simulink library "DelayLibraryBtc"  (R2022b)
settings: Solver=VariableStepAuto  StartTime=0.0  StopTime=10.0  RelTol=1e-3
undefined symbols (not defined in the file or in its folder): Row
libraries: HandyTextFile x6, AudioStats x4, FeaturePath x3, ITC x2, TuneVar x2, CapturedConstLib x1, TOP x1, RTC x1, $bdroot x1
settings Model: Creator=sd49596  LastModifiedBy=jz1055514
settings SolverCC: AlgebraicLoopSolver=TrustRegion
settings DebuggingCC: UnconnectedInputMsg=warning  UnconnectedOutputMsg=warning  UnconnectedLineMsg=warning  SFMachineParentedDataDiag=warning
settings ModelReferenceCC: EnableRefExpFcnMdlSchedulingChecks=on

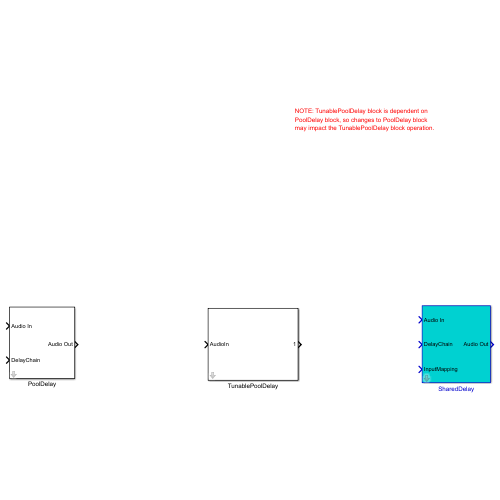
[thumbnail: Simulink's stored preview of the top-level diagram]
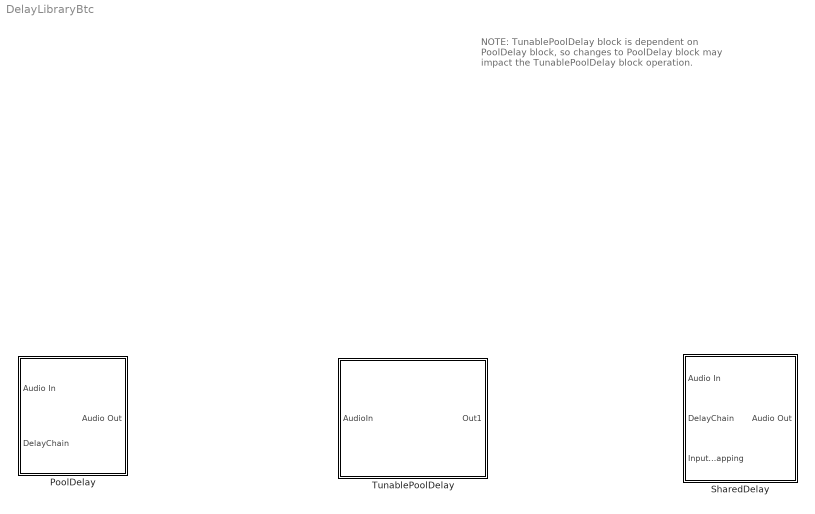
== system DelayLibraryBtc ==
  note: NOTE: TunablePoolDelay block is dependent on
      | PoolDelay block, so changes to PoolDelay block
      | may impact the TunablePoolDelay block operation.
  PoolDelay : Subsystem  mask(Bose Pool Delay){Config=[]}
      mask prompts: Config "PoolDelayConfig"
      mask help:
      | Pool Delay is a multi-channel delay module with one single delay pool and adjustable delays per channel.  It provides support for delays greater than or equal to zero for one or more channels.  Total delay buffer size is the sum of all channel delays.  The Pool Delay model supports three different implementations, selectable from the model mask:
      |
      | - L1 Memory:  Optimized CRL (Code Replacement Library) code running on core with delay buffer in L1 Memory
      | - L2 Memory:  Optimized CRL code running on core and using DMA for memory copies with primary delay buffer in L2 or L3 Memory
      | - Generic:  Generic Matlab implementation running on core for targets without CRL support
      |
      | This model has two inputs and one output:
      |
      | - AudioIn [in]:  Audio input stream containing audio frame samples for one or more channels  [frameSize x numChannels]
      | - Delay [in]:  Delay in samples for each channel  [1 x numChannels]
      | - AudioOut [out]:  Audio output stream containing delayed audio frame samples for one or more channels  [frameSize x numChannels]
      |
      | NOTE: The Pool Delay codeWorkMemory buffer should always be mapped to L1 memory or core MIPS usage will increase.
      |
      | For more information, please see 'Help'.
      mask init:
      | blkh=gcbh;
      | Config=BTConfig.Assert(blkh,Config);
      | 
      | Config.Validate();
      | Config.DoMaskInit(blkh);
      mask Help:
      | Help on Mask Parameters:
      | 
      | All variants of the model contain the following mask parameters:
      | - Implementation:  Selects the desired model implementation to use (L1 Memory, L2 Memory, or Generic)
      | - Total Allotted Delay:  The provides delay buffer sizing for the maximum Room Model Down Load (RMDL) or non-RMDL delay configuration required.  It is the sum of all channels delays in samples for the largest RMDL delay case.  (scalar)
      | - Frame Size:  Specifies the audio frame size in samples (scalar)
      | - Number Channels:  Specifies the number of channel and applies to the audio input, output, and delay channels (scalar)
      | 
      | The 'L2 Memory' implementation contains the following additional mask parameter:
      | 
      | - Delay Sizes Required: The appropriate check boxes must be checked to specify delay categories required.  Delay categories include the following: (delays <= frameSize), (frameSize < delays < (2 * frameSize)), and (delays >= (2 * frameSize).  The correct selection of these delay categories is required to ensure the delay buffers and other model data is sized correctly.
      | 
      | Note that since the 'L2 Memory' implementations takes advantage of DMA memory copies performed by the hardware DMA engine, the implementation differs from the other model implementations and in order to minimize the memory usage required to support all channel delay configurations, the channel delay categories required must be known.  The specific delay cases required for RMDL and non-RMDL model instances determine overall memory required for delay buffers and DMA descriptor memory.
      | 
      | Mask Usage Example:
      | 
      | 3 input and output channels, with channel delays of 16, 48, 80 samples for a case that does not require RMDL, and a frame size of 32 samples.
      | 
      | For example, to use the  L1 Memory implementation, set the mask parameters as follows:
      | 
      | Implementation = 'L1 Memory'
      | Total RMDL Allotted Delay = 144        (16 + 48 + 80)
      | Frame Size = 32
      | Number Channels = 3
      | 
      | For the same example with the L2 Memory implementation, set all the above parameters as stated, except with:
      | 
      | Implementation = 'L2 Memory'
      | Delay Sizes Required should have all delay categories checked, as the delays of 16, 48, 80 include all categories.  These parameters and the Total Allotted Delay are used to size memory to support the delay configuration.  If for example, all delays required were less than equal to a frame only that delay category should be checked.
      | 
      | Note that 'Delay Sizes Required' is specific to the L2 Memory implementation and does not apply to the other implementations.
      | 
      | The 'Generic' implementation would require the identical mask parameter initialization as the L1 memory implementation, except with:
      | 
      | Implementation = 'Generic'
  SharedDelay : Subsystem  mask(Bose Shared Delay){Config=[]}
      mask prompts: Config "SharedDelayConfig"
      mask help:
      | Shared Delay is a multi-input channel delay module with one or more adjustable output delay taps per input channel, based on how input channels are mapped to outputs.  It provides support for delays greater than or equal to zero.  The Shared Delay model supports only one implementation.  It is a DMA based write before delay buffer read implementation, with total delay buffer size of the sum of the maximum output channel tap delay for each input channel, plus one frame size per input channel.
      |
      | This model has two inputs and one output:
      |
      | - AudioIn [in]:  Audio input stream containing audio frame samples for one or more input channels  [frameSize x numInputs]
      | - DelayChain [in]:  Delay in samples for all input channel's output tap channels  [1 x numOutputs]
      | - InputMapping [in]:  Zero based mapping of input channels to output tap channels  [1 x numOutputs]
      | - AudioOut [out]:  Audio output stream containing delayed audio frame samples for one or more output channels  [frameSize x numOutputs]
      |
      | The delay buffer can be mapped to L2 or L3 memory with proper definition of the code generated pragma section memory mappings.
      |
      | NOTE: The Shared Delay codeWorkMemory buffer should always be mapped to L1 memory or core MIPS usage will increase.
      |
      | For more information, please see 'Help'.
      mask init:
      | blkh=gcbh;
      | Config=BTConfig.Assert(blkh,Config);
      | % Validate mask settings
      | Config.Validate();
      | Config.DoMaskInit(blkh);
      mask Help:
      | Help on Mask Parameters:
      | 
      | The Shared Delay model contains the following mask parameters:
      | 
      | - Total Allotted Delay:  Specifies delay buffer sizing for the maximum Room Model Down Load (RMDL) or non-RMDL delay configuration required.  It is the sum of the maximum output channel tap delay for each input channel in samples that supports the largest RMDL delay case.  (scalar)
      | - Frame Size:  Specifies the audio frame size in samples (scalar)
      | - Number Input Channels:  Specifies the number of input channels and applies to the audio inputs (scalar)
      | - Number Output Channels:  Specifies the number of output channels and applies to the audio outputs, delays and input mapping (scalar)
      | 
      | Mask Usage Example:
      | 
      | 2 input channels, with output channel tap delays of 16, 48, 80 samples for input 1 and output channel tap delays of 37, 62 samples for input channel 2.    Assumption is this case does not require RMDL and the frame size is 32 samples.
      | 
      | For this example, set the mask parameters and inputs as follows:
      | 
      | Total Allotted Delay = 142        max( [16 48 80] ) + max( [37  62] ) = 80 + 62
      | Frame Size = 32
      | Number Inputs = 2
      | Number Outputs = 5                (3 + 2)
      | 
      | DelayChain = [16 48 80 37 62]
      | InputMapping = [0 0 0 1 1]
  TunablePoolDelay : Subsystem  mask{Config=[]}
      mask prompts: Config "TunablePoolDelayConfig"
      mask init:
      | blkh=gcbh;
      | Config=BTConfig.Assert(blkh,Config);
      | 
      | Config.Validate();
      | Config.DoMaskInit(blkh);

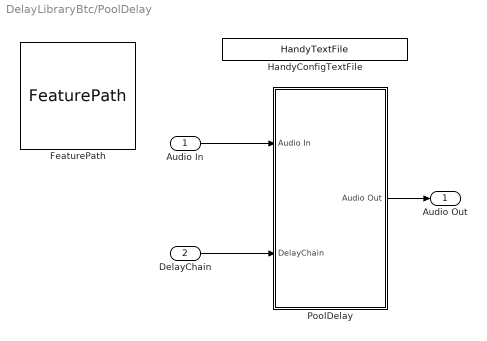
== system DelayLibraryBtc/PoolDelay ==
  Audio In : Inport
  DelayChain : Inport  Port=2  OutDataTypeStr=uint32  PortDimensions=[1, Config.NumChannels]
  FeaturePath : FeaturePath/FeaturePath  FeatureName=PoolDelay  IsGroup=off  GroupNumber=-1  IsModule=off  TriggerInit=[-40 9 75 116]
      settings: SourceProductName=Bose Talaria
  HandyConfigTextFile : HandyTextFile/HandyTextFile  TemplateSource=Config  FileSuffix=File  OpenDialogOnLoad=off  UseThisBlockName=off  AddGrandParentNamePrefix=off  TheDefaultText=% $(FILENAME) $(PREFIX) $(SUFFIX)  ShowInLibBrowser=on
      settings: SourceProductName=Bose Talaria
  PoolDelay : Subsystem  Variant=on
  Audio Out : Outport
  wires:
  Audio In/1 -> PoolDelay/1(Audio In)
  DelayChain/1 -> PoolDelay/2(DelayChain)
  PoolDelay/1(Audio Out) -> Audio Out/1

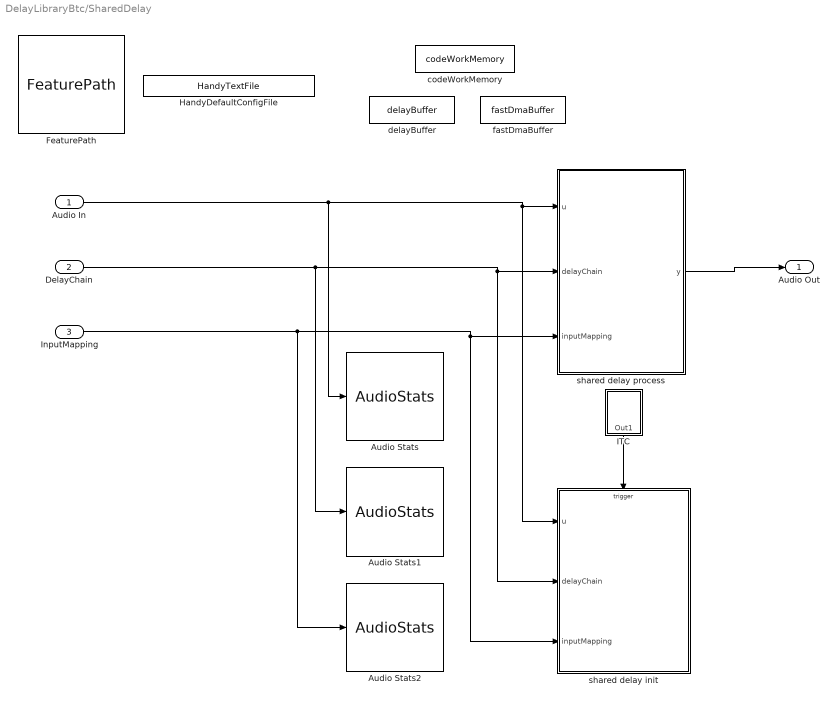
== system DelayLibraryBtc/SharedDelay ==
  Audio In : Inport
  DelayChain : Inport  Port=2  OutDataTypeStr=int32  PortDimensions=[1, Config.NumOutputs]
  InputMapping : Inport  Port=3  OutDataTypeStr=int32  PortDimensions=[1 Config.NumOutputs]
  Audio Stats : AudioStats/AudioStats  DoSampleRate=off  TypeSampleRate=Inherit: auto  DoCallRate=off  TypeCallRate=Inherit: auto  DoFrameSize=off  TypeFrameSize=Inherit: auto  DoChannelCount=off  TypeChannelCount=Inherit: auto  DoTaskRateFactor=off  TypeTaskRateFactor=Inherit: auto  MacroNameRoot=AUDIO  MacroNameRootEval='AUDIO'  IsMacroNameEval=off  MacroSampleRate=off  MacroCallRate=off  MacroFrameSize=off  MacroChannelCount=off  MacroTaskRateFactor=off  MacroTaskId=off  ValidateSampleRate=off  ValueSampleRate=[]  ValidateCallRate=off  ValueCallRate=[]  ValidateFrameSize=on  ValueFrameSize=Config.FrameSize  ValidateChannelCount=on  ValueChannelCount=Config.NumInputs  ValidateTaskRateFactor=off  ValueTaskRateFactor=[]
      settings: SourceProductName=Bose Talaria
  Audio Stats1 : AudioStats/AudioStats  DoSampleRate=off  TypeSampleRate=Inherit: auto  DoCallRate=off  TypeCallRate=Inherit: auto  DoFrameSize=off  TypeFrameSize=Inherit: auto  DoChannelCount=off  TypeChannelCount=Inherit: auto  DoTaskRateFactor=off  TypeTaskRateFactor=Inherit: auto  MacroNameRoot=AUDIO  MacroNameRootEval='AUDIO'  IsMacroNameEval=off  MacroSampleRate=off  MacroCallRate=off  MacroFrameSize=off  MacroChannelCount=off  MacroTaskRateFactor=off  MacroTaskId=off  ValidateSampleRate=off  ValueSampleRate=[]  ValidateCallRate=off  ValueCallRate=[]  ValidateFrameSize=off  ValueFrameSize=[]  ValidateChannelCount=on  ValueChannelCount=Config.NumOutputs  ValidateTaskRateFactor=off  ValueTaskRateFactor=[]
      settings: SourceProductName=Bose Talaria
  Audio Stats2 : AudioStats/AudioStats  DoSampleRate=off  TypeSampleRate=Inherit: auto  DoCallRate=off  TypeCallRate=Inherit: auto  DoFrameSize=off  TypeFrameSize=Inherit: auto  DoChannelCount=off  TypeChannelCount=Inherit: auto  DoTaskRateFactor=off  TypeTaskRateFactor=Inherit: auto  MacroNameRoot=AUDIO  MacroNameRootEval='AUDIO'  IsMacroNameEval=off  MacroSampleRate=off  MacroCallRate=off  MacroFrameSize=off  MacroChannelCount=off  MacroTaskRateFactor=off  MacroTaskId=off  ValidateSampleRate=off  ValueSampleRate=[]  ValidateCallRate=off  ValueCallRate=[]  ValidateFrameSize=off  ValueFrameSize=[]  ValidateChannelCount=on  ValueChannelCount=Config.NumOutputs  ValidateTaskRateFactor=off  ValueTaskRateFactor=[]
      settings: SourceProductName=Bose Talaria
  FeaturePath : FeaturePath/FeaturePath  FeatureName=SharedDelay  IsGroup=off  GroupNumber=-1  IsModule=off  TriggerInit=[185 -31 300 76]
      settings: SourceProductName=Bose Talaria
  HandyDefaultConfigFile : HandyTextFile/HandyTextFile  TemplateSource=Config  FileSuffix=Init  OpenDialogOnLoad=off  UseThisBlockName=off  AddGrandParentNamePrefix=off  TheDefaultText=|  ShowInLibBrowser=on
      | % $(FILENAME) Setup model parameters for each "Init" callback (e.g. update diagram)
      | sample_rate_in_hertz = 44100;
      | frame_size = 32;
      | sysin_channel_count = 2;
      settings: SourceProductName=Bose Talaria
  ITC : Subsystem  mask(Bose Initialization Trigger Control){}
      mask help: This block emits a function trigger for logic intended to execute at subsystem initialization time. Make sure not to reference any "live" signals
      mask init:
      | CodeID = InitTriggerControlMask.DoInit(gcbh);
      | ok = true;
      mask Display:
      | % retrieve icon definition
      | [path,w,h] = InitTriggerControlMask.Icon();
      | 
      | % retrieve the block's pixel size
      | pos = get(gcbh,'position');
      | bw = pos(3) - pos(1);
      | bh = pos(4) - pos(2);
      | 
      | % draw  icon to the center left
      | xAdj = bw/2 - w/2;
      | yAdj = bh/2 - h/2 + 4;
      | for i=1:length(path)
      |     patch(path(i).x+xAdj, path(i).y+yAdj, path(i).rgb);
      | end
      | 
      | text(bw*0.5, bh*0.2, 'ITC', 'horizontalAlignment', 'center');
      | 
      | % show X on error
      | if (exist('ok','var') && ok)
      | 	patch(0,0,[1 1 1]);
      | 	patch(bw,bh,[1 1 1]);
      | else
      | 	tx=bw*0.03;
      | 	ty=bh*0.03;
      | 	patch([0 tx bw bw-tx], [ty 0 bh-ty bh], [1 0 0]);
      | 	patch([0 bw-tx bw tx], [bh-ty 0 ty bh], [1 0 0]);
      | end
  codeWorkMemory : DataStoreMemory  DataStoreName=codeWorkMemory  WriteAfterWriteMsg=warning  InitialValue=Config.CodeWorkMemoryInitVal  EmbeddedSignalClassName=Blocklib.Signal  ShowAdditionalParam=off  OutDataTypeStr=uint32
  delayBuffer : DataStoreMemory  DataStoreName=delayBuffer  ReadBeforeWriteMsg=warning  WriteAfterWriteMsg=warning  WriteAfterReadMsg=warning  InitialValue=Config.DelayBufferInitVal  EmbeddedSignalClassName=Blocklib.Signal  ShowAdditionalParam=off  OutDataTypeStr=single
  fastDmaBuffer : DataStoreMemory  DataStoreName=fastDmaBuffer  ReadBeforeWriteMsg=warning  WriteAfterWriteMsg=warning  WriteAfterReadMsg=warning  InitialValue=Config.FastDelayBufferInitVal  EmbeddedSignalClassName=Blocklib.Signal  ShowAdditionalParam=off  OutDataTypeStr=single
  shared delay init : MATLAB Function  TreatAsAtomicUnit=on  RTWFcnName=foo
  shared delay process : MATLAB Function  TreatAsAtomicUnit=on
  Audio Out : Outport  VectorParamsAs1DForOutWhenUnconnected=off
  wires:
  Audio In/1 -> shared delay process/1(u), shared delay init/1(u), Audio Stats/1
  InputMapping/1 -> shared delay process/3(inputMapping), shared delay init/3(inputMapping), Audio Stats2/1
  ITC/1(Out1) -> shared delay init/Trigger
  shared delay process/1(y) -> Audio Out/1
  DelayChain/1 -> shared delay process/2(delayChain), shared delay init/2(delayChain), Audio Stats1/1

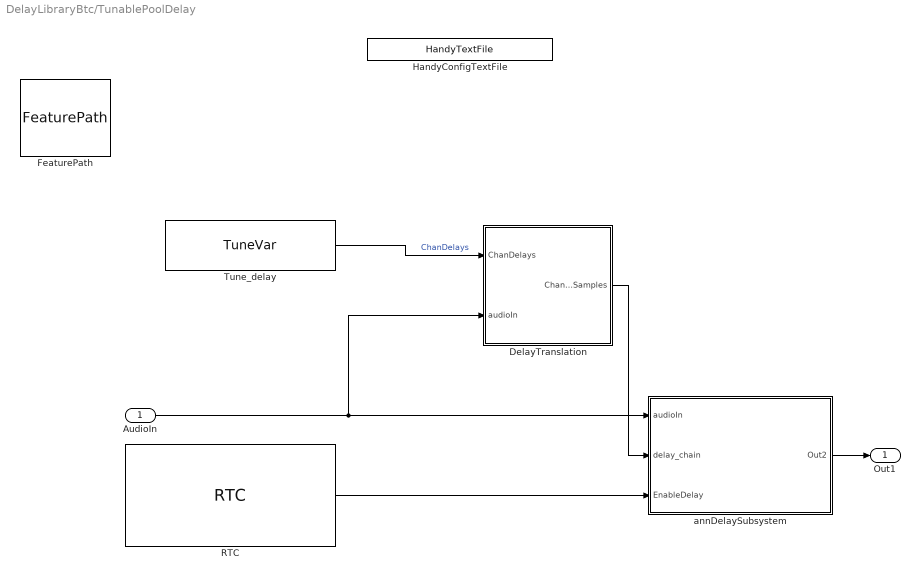
== system DelayLibraryBtc/TunablePoolDelay ==
  AudioIn : Inport
  DelayTranslation : Subsystem  mask{delayType=Config.delayType, maxTotalDelay=Config.MaxTotalDelay}
      mask prompts: delayType "Delay Type"; maxTotalDelay "Max Total Delay"
  FeaturePath : FeaturePath/FeaturePath  FeatureName=TunablePoolDelay  IsGroup=off  GroupNumber=-1  IsModule=off  TriggerInit=[500 209 590 286]
      settings: SourceProductName=Bose Talaria
  HandyConfigTextFile : HandyTextFile/HandyTextFile  TemplateSource=Config  FileSuffix=File  OpenDialogOnLoad=off  UseThisBlockName=off  AddGrandParentNamePrefix=off  TheDefaultText=% $(FILENAME) $(PREFIX) $(SUFFIX)  ShowInLibBrowser=on
      settings: SourceProductName=Bose Talaria
  RTC : RTC/RTC  REQ_Priority=RTC_Mask.NormalPriority  RequestAtInit=off  EnableRequest=off  REQElemName1=Enable_annDelay  REQElemType1=uint32  REQElemWidth1=1  REQElemInitial1=Config.enableDelay  REQElemType2=uint32  REQElemWidth2=1  REQElemInitial2=[]  REQElemType3=uint32  REQElemWidth3=1  REQElemInitial3=[]  REQElemType4=uint32  REQElemWidth4=1  REQElemInitial4=[]  REQElemType5=uint32  REQElemWidth5=1  REQElemInitial5=[]  REQElemType6=uint32  REQElemWidth6=1  REQElemInitial6=[]  REQElemType7=uint32  REQElemWidth7=1  REQElemInitial7=[]  REQElemType8=uint32  REQElemWidth8=1  REQElemInitial8=[]  REQElemType9=uint32  REQElemWidth9=1  REQElemInitial9=[]  REQElemType10=uint32  REQElemWidth10=1  REQElemInitial10=[]  EnableResponse=on  EnableRSP_StatusIn=off  RSPElemType1=uint32  RSPElemWidth1=1  RSPElemType2=uint32  RSPElemWidth2=1  RSPElemType3=uint32  RSPElemWidth3=1  RSPElemType4=uint32  RSPElemWidth4=1  RSPElemType5=uint32  RSPElemWidth5=1  RSPElemType6=uint32  RSPElemWidth6=1  RSPElemType7=uint32  RSPElemWidth7=1  RSPElemType8=uint32  RSPElemWidth8=1  RSPElemType9=uint32  RSPElemWidth9=1  RSPElemType10=uint32  RSPElemWidth10=1  EnableNotification=off  EnableNTF_PrepTrig=off  NTFElemType1=uint32  NTFElemWidth1=1  NTFElemType2=uint32  NTFElemWidth2=1  NTFElemType3=uint32  NTFElemWidth3=1  NTFElemType4=uint32  NTFElemWidth4=1  NTFElemType5=uint32  NTFElemWidth5=1  NTFElemType6=uint32  NTFElemWidth6=1  NTFElemType7=uint32  NTFElemWidth7=1  NTFElemType8=uint32  NTFElemWidth8=1  NTFElemType9=uint32  NTFElemWidth9=1  NTFElemType10=uint32  NTFElemWidth10=1  MaskMessageName=Enable_Delay
      settings: SourceProductName=Bose Talaria
  Tune_delay : TuneVar/TuneVar  TuneName=ChanDelays  SpecifyMaxSize=off  VariableDim=1 (Row)  MaxSize=[1 1]  TunabilityNumber=1  MinValue=[]  MaxValue=[]  TriggerInit=[645 350 815 400]  MaskValue=Config.delayChains
      settings: SourceProductName=Bose Talaria
  annDelaySubsystem : Subsystem
  Out1 : Outport  VectorParamsAs1DForOutWhenUnconnected=off
  wires:
  AudioIn/1 -> DelayTranslation/2(audioIn), annDelaySubsystem/1(audioIn)
  RTC/1 -> annDelaySubsystem/3(EnableDelay)
  Tune_delay/1 -> DelayTranslation/1(ChanDelays)  "ChanDelays"
  annDelaySubsystem/1(Out2) -> Out1/1
  DelayTranslation/1(ChanDelaysSamples) -> annDelaySubsystem/2(delay_chain)

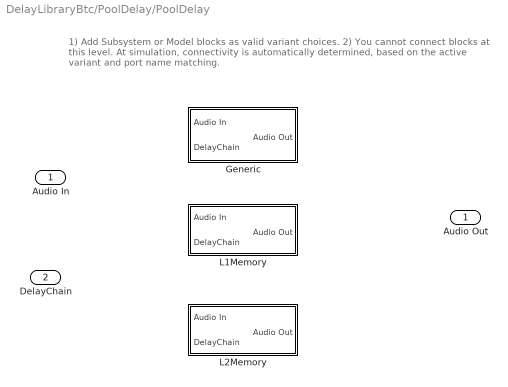
== system DelayLibraryBtc/PoolDelay/PoolDelay ==
  note: 1) Add Subsystem or Model blocks as valid variant choices.
      | 2) You cannot connect blocks at this level. At simulation, connectivity is automatically
      | determined, based on the active variant and port name matching.
  Audio In : Inport
  DelayChain : Inport  Port=2
  Generic : Subsystem  VariantControl=(default)
  L1Memory : Subsystem  VariantControl=Config.Breed == PoolDelayBreedEnum.L1Memory
  L2Memory : Subsystem  VariantControl=Config.Breed == PoolDelayBreedEnum.L2Memory
  Audio Out : Outport

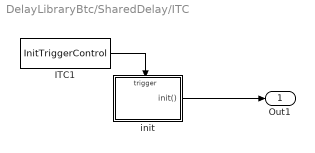
== system DelayLibraryBtc/SharedDelay/ITC ==
  ITC1 : S-Function  FunctionName=InitTriggerControl  Parameters=CodeID, 0  SFunctionDeploymentMode=off  EnableBusSupport=off
  init : MATLAB Function  TreatAsAtomicUnit=on  RTWFcnName=InitTrigger_DelayLibraryBtc_1_62
      settings: RTWSystemCode=Nonreusable function
  Out1 : Outport  VectorParamsAs1DForOutWhenUnconnected=off
  wires:
  init/1(init()) -> Out1/1
  ITC1/1 -> init/Trigger

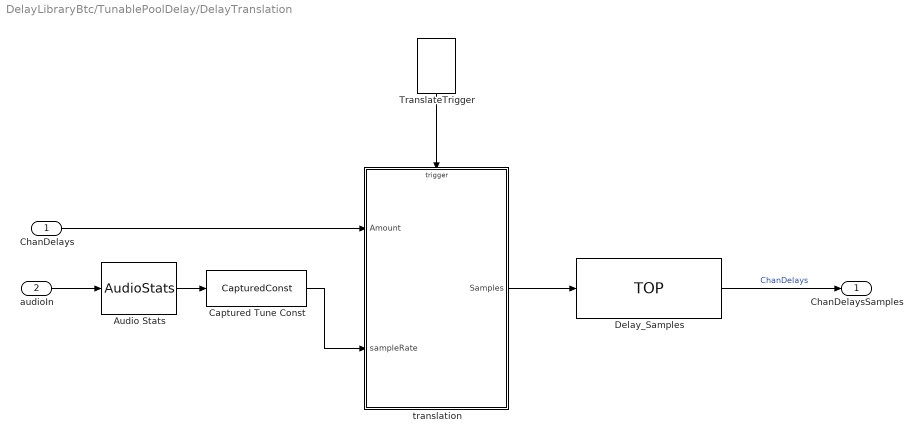
== system DelayLibraryBtc/TunablePoolDelay/DelayTranslation ==
  ChanDelays : Inport
  audioIn : Inport  Port=2
  Audio Stats : AudioStats/AudioStats  DoSampleRate=on  TypeSampleRate=Inherit: auto  DoCallRate=off  TypeCallRate=Inherit: auto  DoFrameSize=off  TypeFrameSize=Inherit: auto  DoChannelCount=off  TypeChannelCount=Inherit: auto  DoTaskRateFactor=off  TypeTaskRateFactor=Inherit: auto  MacroNameRoot=AUDIO  MacroNameRootEval='AUDIO'  IsMacroNameEval=off  MacroSampleRate=off  MacroCallRate=off  MacroFrameSize=off  MacroChannelCount=off  MacroTaskRateFactor=off  MacroTaskId=off  ValidateSampleRate=off  ValueSampleRate=[]  ValidateCallRate=off  ValueCallRate=[]  ValidateFrameSize=off  ValueFrameSize=[]  ValidateChannelCount=off  ValueChannelCount=[]  ValidateTaskRateFactor=off  ValueTaskRateFactor=[]
      settings: SourceProductName=Bose Talaria
  Captured Tune Const : CapturedConstLib/CapturedConst  TriggerInit=[1245 262 1345 298]  Role=Automatic
      settings: SourceProductName=Bose Talaria
  Delay_Samples : TOP/TOP  TriggerInit=[575 240 720 300]  TopName=ChanDelays  DataTypeOut=uint32  BankNumber=0  PreOverlay=false  PostOverlay=Config.PostOverlayRequired  CompatibilityString=[]  Role=Automatic
      settings: SourceProductName=Bose Talaria
  TranslateTrigger : TuneVar/TranslateTrigger  TriggerInit=[1456 30 1494 85]
      settings: SourceProductName=Bose Talaria
  translation : MATLAB Function  TreatAsAtomicUnit=on
  ChanDelaysSamples : Outport  VectorParamsAs1DForOutWhenUnconnected=off
  wires:
  ChanDelays/1 -> translation/1(Amount)
  Audio Stats/1 -> Captured Tune Const/1
  TranslateTrigger/1 -> translation/Trigger
  audioIn/1 -> Audio Stats/1
  Delay_Samples/1 -> ChanDelaysSamples/1  "ChanDelays"
  Captured Tune Const/1 -> translation/2(sampleRate)
  translation/1(Samples) -> Delay_Samples/1

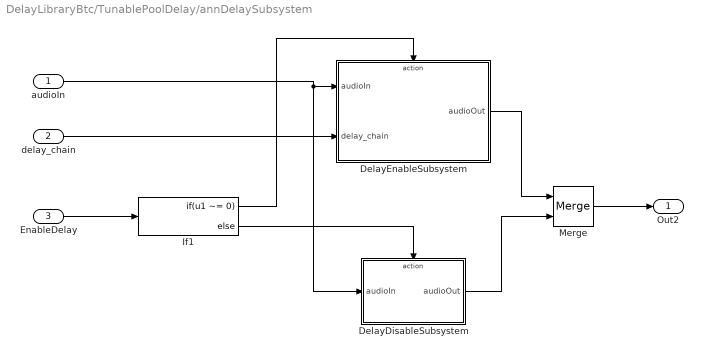
== system DelayLibraryBtc/TunablePoolDelay/annDelaySubsystem ==
  audioIn : Inport
  delay_chain : Inport  Port=2
  EnableDelay : Inport  Port=3
  DelayDisableSubsystem : Subsystem  TreatAsAtomicUnit=on
  DelayEnableSubsystem : Subsystem  TreatAsAtomicUnit=on
  If1 : If  IfExpression=u1 ~= 0
  Merge : Merge
  Out2 : Outport  VectorParamsAs1DForOutWhenUnconnected=off
  wires:
  If1/1 -> DelayEnableSubsystem/Action
  audioIn/1 -> DelayEnableSubsystem/1(audioIn), DelayDisableSubsystem/1(audioIn)
  EnableDelay/1 -> If1/1
  If1/2 -> DelayDisableSubsystem/Action
  DelayEnableSubsystem/1(audioOut) -> Merge/1
  delay_chain/1 -> DelayEnableSubsystem/2(delay_chain)
  DelayDisableSubsystem/1(audioOut) -> Merge/2
  Merge/1 -> Out2/1

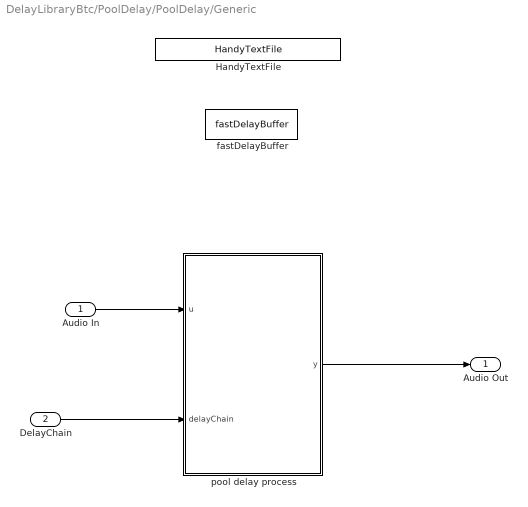
== system DelayLibraryBtc/PoolDelay/PoolDelay/Generic ==
  Audio In : Inport
  DelayChain : Inport  Port=2
  HandyTextFile : HandyTextFile/HandyTextFile  TemplateSource=<dialog fields>  FileSuffix=BreedConfig  OpenDialogOnLoad=off  UseThisBlockName=off  AddGrandParentNamePrefix=on  TheDefaultText=% $(FILENAME) $(PREFIX) $(SUFFIX)  ShowInLibBrowser=on
      settings: SourceProductName=Bose Talaria
  fastDelayBuffer : DataStoreMemory  DataStoreName=fastDelayBuffer  ReadBeforeWriteMsg=warning  WriteAfterWriteMsg=warning  WriteAfterReadMsg=warning  InitialValue=Config.BreedObj.FastDelayBufferInitVal  ShowAdditionalParam=off  OutDataTypeStr=single
  pool delay process : MATLAB Function  TreatAsAtomicUnit=on
  Audio Out : Outport
  wires:
  DelayChain/1 -> pool delay process/2(delayChain)
  Audio In/1 -> pool delay process/1(u)
  pool delay process/1(y) -> Audio Out/1

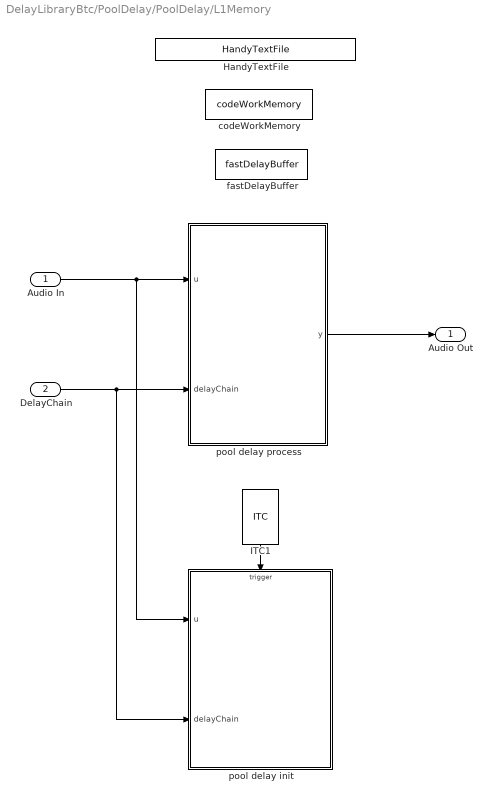
== system DelayLibraryBtc/PoolDelay/PoolDelay/L1Memory ==
  Audio In : Inport
  DelayChain : Inport  Port=2
  HandyTextFile : HandyTextFile/HandyTextFile  TemplateSource=<dialog fields>  FileSuffix=BreedConfig  OpenDialogOnLoad=off  UseThisBlockName=off  AddGrandParentNamePrefix=on  TheDefaultText=% $(FILENAME) $(PREFIX) $(SUFFIX)  ShowInLibBrowser=on
      settings: SourceProductName=Bose Talaria
  ITC1 : ITC/ITC
      settings: SourceProductName=Bose Talaria
  codeWorkMemory : DataStoreMemory  DataStoreName=codeWorkMemory  WriteAfterWriteMsg=warning  InitialValue=Config.BreedObj.CodeWorkMemoryInitVal  ShowAdditionalParam=off  OutDataTypeStr=uint32
  fastDelayBuffer : DataStoreMemory  DataStoreName=fastDelayBuffer  ReadBeforeWriteMsg=warning  WriteAfterWriteMsg=warning  WriteAfterReadMsg=warning  InitialValue=Config.BreedObj.FastDelayBufferInitVal  ShowAdditionalParam=off  OutDataTypeStr=single
  pool delay init : MATLAB Function  TreatAsAtomicUnit=on  RTWFcnName=foo
  pool delay process : MATLAB Function  TreatAsAtomicUnit=on
  Audio Out : Outport
  wires:
  Audio In/1 -> pool delay init/1(u), pool delay process/1(u)
  DelayChain/1 -> pool delay init/2(delayChain), pool delay process/2(delayChain)
  pool delay process/1(y) -> Audio Out/1
  ITC1/1 -> pool delay init/Trigger

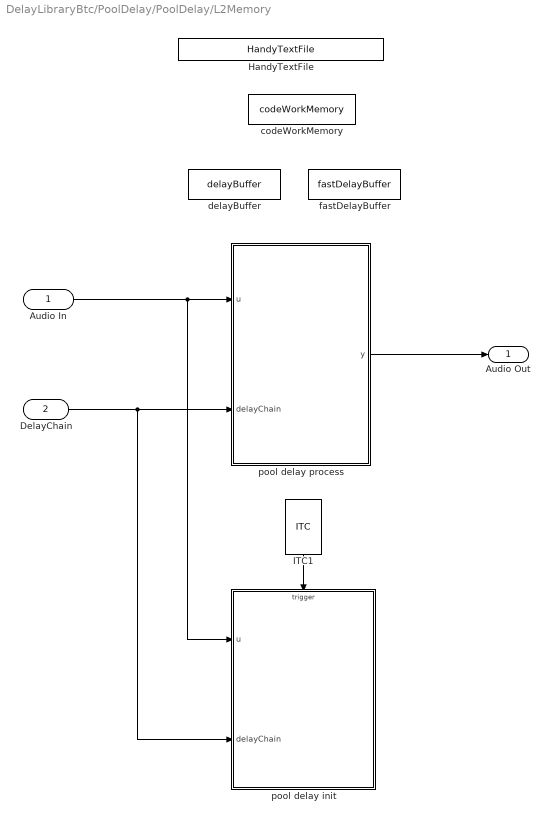
== system DelayLibraryBtc/PoolDelay/PoolDelay/L2Memory ==
  Audio In : Inport
  DelayChain : Inport  Port=2
  HandyTextFile : HandyTextFile/HandyTextFile  TemplateSource=<dialog fields>  FileSuffix=BreedConfig  OpenDialogOnLoad=off  UseThisBlockName=off  AddGrandParentNamePrefix=on  TheDefaultText=% $(FILENAME) $(PREFIX) $(SUFFIX)  ShowInLibBrowser=on
      settings: SourceProductName=Bose Talaria
  ITC1 : ITC/ITC
      settings: SourceProductName=Bose Talaria
  codeWorkMemory : DataStoreMemory  DataStoreName=codeWorkMemory  WriteAfterWriteMsg=warning  InitialValue=Config.BreedObj.CodeWorkMemoryInitVal  ShowAdditionalParam=off  OutDataTypeStr=uint32
  delayBuffer : DataStoreMemory  DataStoreName=delayBuffer  ReadBeforeWriteMsg=warning  WriteAfterWriteMsg=warning  WriteAfterReadMsg=warning  InitialValue=Config.BreedObj.DelayBufferInitVal  ShowAdditionalParam=off  OutDataTypeStr=single
  fastDelayBuffer : DataStoreMemory  DataStoreName=fastDelayBuffer  ReadBeforeWriteMsg=warning  WriteAfterWriteMsg=warning  WriteAfterReadMsg=warning  InitialValue=Config.BreedObj.FastDelayBufferInitVal  ShowAdditionalParam=off  OutDataTypeStr=single
  pool delay init : MATLAB Function  TreatAsAtomicUnit=on  RTWFcnName=foo
  pool delay process : MATLAB Function  TreatAsAtomicUnit=on
  Audio Out : Outport
  wires:
  pool delay process/1(y) -> Audio Out/1
  Audio In/1 -> pool delay init/1(u), pool delay process/1(u)
  DelayChain/1 -> pool delay init/2(delayChain), pool delay process/2(delayChain)
  ITC1/1 -> pool delay init/Trigger

== system DelayLibraryBtc/TunablePoolDelay/annDelaySubsystem/DelayDisableSubsystem ==
  audioIn : Inport
  Action Port : ActionPort  ActionPortLabel=else
  audioOut : Outport  VectorParamsAs1DForOutWhenUnconnected=off
  wires:
  audioIn/1 -> audioOut/1

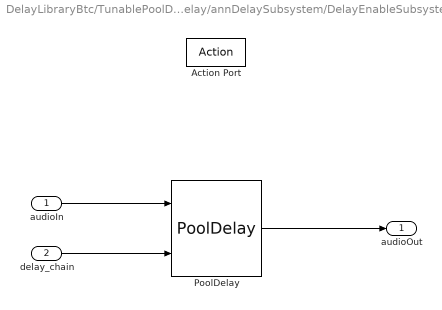
== system DelayLibraryBtc/TunablePoolDelay/annDelaySubsystem/DelayEnableSubsystem ==
  audioIn : Inport
  delay_chain : Inport  Port=2
  Action Port : ActionPort  ActionPortLabel=if(u1 ~= 0)
  PoolDelay : $bdroot/PoolDelay  Config=Config.poolDelay
  audioOut : Outport  VectorParamsAs1DForOutWhenUnconnected=off
  wires:
  PoolDelay/1 -> audioOut/1
  audioIn/1 -> PoolDelay/1
  delay_chain/1 -> PoolDelay/2

== matlab function DelayLibraryBtc/PoolDelay/PoolDelay/L1Memory/pool delay init ==
  data: u input; delayChain input; codeWorkMemory data_store_memory; fastDelayBuffer data_store_memory
  events: trigger input FUNCTION_CALL_EVENT
function pool_delay_init(u, delayChain)

% Pool delay function provides delay lines for N channels.  Core
% implementation provides delay of any positive integer value. 
% 
% Parameters:
%   u:              Input channels [frame size x number of inputs]
%   delayChain:     Delay in samples for each channel [1 x delay per channel]
%
% Global parameters:
%   fastDelayBuffer: Fast delay line circular buffer containing all channel  
%                    delay state data
%   codeWorkMemory: Working memory set up during roommode reset/init CRL
%                   function call [1 x codeWorkMemorySize]

% Extract configuration information from inut
[frameSize, numChannels]  = size(u);

global fastDelayBuffer;
global codeWorkMemory;

% Get the work memory and delay buffer sizes
workMemorySize = numel(codeWorkMemory);
fastDelayBufferSize = numel(fastDelayBuffer);

% Set correct data types
frameSize = uint32(frameSize);
numChannels = uint32(numChannels);
delayChain = uint32(delayChain);
workMemorySize = uint32(workMemorySize);
fastDelayBufferSize = uint32(fastDelayBufferSize);
    
y = pool_delay_core_init(u, fastDelayBuffer, fastDelayBufferSize, ...
                         delayChain, numChannels, frameSize, ...
                         codeWorkMemory, workMemorySize);

                         
% NOTE: The CRL mechanism requires an output for the function call,
% and appears to be optimized out if that return value isn't used. 
% This is a dummy operation to make sure CRL ends up in generated code
codeWorkMemory(1) = y; 
end

% Pool delay CRL core initialization function conceptual specification  
function y = pool_delay_core_init(u, fastDelayBuffer, fastDelayBufferSize, ... 
                                  delayChain, numChannels, frameSize, ...
                                  workMemory, workMemorySize)
% If target == codegen, error out if no CRL found
coder.replace('-errorifnoreplacement');

% No init simulation code, but need to do something to ensure CRL does not
% get optimized out
y = single(workMemory(1) + 1);

end

== matlab function DelayLibraryBtc/PoolDelay/PoolDelay/L1Memory/pool delay process ==
  data: u input; delayChain input; y output; codeWorkMemory data_store_memory; fastDelayBuffer data_store_memory
function y = pool_delay_process(u, delayChain)
% Pool delay function provides delay lines for N channels.  Core
% implementation provides delay of any positive integer value.
%
% Parameters:
%   u:              Input channels [frame size x number of inputs]
%   delayChain:     Delay in samples for each channel [1 x delay per channel]
%
% Global parameters:
%   fastDelayBuffer: Fast delay line circular buffer containing all channel  
%                    delay state data
%   codeWorkMemory:  Working memory set up during roommode reset/init CRL
%                    function call [1 x codeWorkMemorySize]

global fastDelayBuffer;
global codeWorkMemory;

% Get the fast delay buffer sizes
fastDelayBufferSize = numel(fastDelayBuffer);

% Set correct data types
delayChain = uint32(delayChain);
fastDelayBufferSize = uint32(fastDelayBufferSize);

% Simulation
if(coder.target('MATLAB') || coder.target('Sfun')) 
        y = PoolDelaySim(u, delayChain, fastDelayBufferSize); 
else
        y = pool_delay_core_process(u, delayChain, codeWorkMemory);
end
end

% Pool delay CRL core step/process function conceptual specification
function y = pool_delay_core_process(u, delayChain, workMemory)
% If target == codegen, error out if no CRL found
coder.replace('-errorifnoreplacement');

[frameSize, numChannels] = size(u);
y = single(zeros(frameSize, numChannels));
end

== matlab function DelayLibraryBtc/SharedDelay/ITC/init ==
  events: trigger input FUNCTION_CALL_EVENT; init output FUNCTION_CALL_EVENT
function init

init();

== matlab function DelayLibraryBtc/TunablePoolDelay/DelayTranslation/translation ==
  data: Samples output; Amount input; sampleRate input; maxTotalDelay parameter; delayType parameter
  events: trigger input FUNCTION_CALL_EVENT
function Samples = fcn(Amount, sampleRate, maxTotalDelay, delayType)

if (delayType == 1) % delay in samples
    Samples = uint32(ceil(Amount.Value));
else % delay in milliseconds
    Samples = uint32(ceil(Amount.Value * 1e-3 * sampleRate));
end

% Check if Channel Delay is greater than max allowed pool delay
chanDelay = uint32(sum(Samples));
if (chanDelay > maxTotalDelay)
    TranslateError('Total delay is bigger than allotted delay');
end

== matlab function DelayLibraryBtc/SharedDelay/shared delay init ==
  data: u input; delayChain input; inputMapping input; codeWorkMemory data_store_memory; delayBuffer data_store_memory; fastDmaBuffer data_store_memory
  events: trigger input FUNCTION_CALL_EVENT
function shared_delay_init(u, delayChain, inputMapping)
% Shared delay function provides multiple delay line tap outputs for each 
% input channel. 
% 
% Parameters:
%   u:               Input channels [frame size x number of inputs]
%   delayChain:      Delay in samples for each channel [1 x number of outputs]
%   inputMapping:    Zero-based input mapping for each filter [1 x number of outputs]
%
% Global parameters:
%   delayBuffer:     Delay line circular buffer containing all channel  
%                    delay state data
%   fastDmaBuffer:   Fast DMA buffer containing all channel outputs for
%                    next frame
%   codeWorkMemory:  Working memory set up during roommode reset/init CRL
%                    function call [1 x codeWorkMemorySize]
%   RMDLshutdown:    Flag to indicate RMDL is in progress [1 x 1]

global delayBuffer;
global fastDmaBuffer;
global codeWorkMemory;

% Extract configuration information from input
[frameSize, numInputs]  = size(u);
numOutputs = numel(delayChain);

% Get the work memory and delay buffer sizes
workMemorySize = numel(codeWorkMemory);
delayBufferSize = numel(delayBuffer);
fastDmaBufferSize = numel(fastDmaBuffer);

% Set correct data types
frameSize = int32(frameSize);
numInputs = int32(numInputs);
numOutputs = int32(numOutputs);
delayChain = int32(delayChain);
inputMapping = int32(inputMapping);
workMemorySize = int32(workMemorySize);
delayBufferSize = int32(delayBufferSize);
fastDmaBufferSize = int32(fastDmaBufferSize);

% Initialization
y = shared_delay_mdma_init(u, delayBuffer, delayBufferSize, ...
                           fastDmaBuffer, fastDmaBufferSize, ...
                           delayChain, inputMapping, numInputs, ... 
                           numOutputs, frameSize, codeWorkMemory, ...
                           workMemorySize);

% NOTE: The CRL mechanism requires an output for the function call,
% and appears to be optimized out if that return value isn't used. 
% This is a dummy operation to make sure CRL ends up in generated code
codeWorkMemory(1) = y; 

end


% Shared delay CRL initialization function conceptual specification
function y = shared_delay_mdma_init(u, delayBuffer, delayBufferSize, ...
                                    fastDmaBuffer, fastDmaBufferSize, ...    
                                    delayChain, inputMapping, numInputs, ...
                                    numOutputs, frameSize, workMemory, ...
                                    workMemorySize) 
% If target == codegen, error out if no CRL found
coder.replace('-errorifnoreplacement');

% No init simulation code, but need to do something to ensure CRL does not
% get optimized out
y = single(workMemory(1) + 1);

end

== matlab function DelayLibraryBtc/SharedDelay/shared delay process ==
  data: u input; delayChain input; inputMapping input; y output; codeWorkMemory data_store_memory; delayBuffer data_store_memory
function y = shared_delay_process(u, delayChain, inputMapping)
% Shared delay function provides multiple delay line tap outputs for each 
% input channel.   
%
% Parameters:
%   u:              Input channels [frame size x number of inputs]
%   delayChain:     Delay in samples for each channel [1 x number of outputs]
%   inputMapping:   Zero-based input mapping for each filter [1 x number of outputs]
%
% Global parameters:
%   delayBuffer:     Delay line circular buffer containing all channel  
%                    delay state data
%   codeWorkMemory:  Working memory set up during roommode reset/init CRL
%                    function call [1 x codeWorkMemorySize]

global delayBuffer;
global codeWorkMemory;

% Get the fast delay buffer sizes
delayBufferSize = numel(delayBuffer);

% Set correct data types
delayChain = int32(delayChain);
delayBufferSize = int32(delayBufferSize);

% Simulation
if(coder.target('MATLAB') || coder.target('Sfun'))
    
    y = SharedDelaySim(u, delayChain, inputMapping, delayBufferSize);        
    
% Code generation
else 
    
    y = shared_delay_mdma_process(u, delayChain, codeWorkMemory);

end

end


% Shared delay CRL step/process function conceptual specification
function y = shared_delay_mdma_process(u, delayChain, workMemory)
% If target == codegen, error out if no CRL found
coder.replace('-errorifnoreplacement');

[frameSize, ~] = size(u);
numOutputs = numel(delayChain);
y = single(zeros(frameSize, numOutputs));
end

== matlab function DelayLibraryBtc/PoolDelay/PoolDelay/L2Memory/pool delay init ==
  data: u input; delayChain input; codeWorkMemory data_store_memory; delayBuffer data_store_memory; fastDelayBuffer data_store_memory
  events: trigger input FUNCTION_CALL_EVENT
function pool_delay_init(u, delayChain)

% Pool delay function provides delay lines for N channels.MDMA
% implementation provides integer value delays of a frame or greater. 
% 
% Parameters:
%   u:              Input channels [frame size x number of inputs]
%   delayChain:     Delay in samples for each channel [1 x delay per channel]
%
% Global parameters:
%   delayBuffer:    Delay line circular buffer containing all channel  
%                   delay state data
%   fastDelayBuffer: Fast delay line circular buffer containing all channel  
%                    delay state data
%   codeWorkMemory: Working memory set up during roommode reset/init CRL
%                   function call [1 x codeWorkMemorySize]

% Extract configuration information from inut
[frameSize, numChannels]  = size(u);

global delayBuffer;
global fastDelayBuffer;
global codeWorkMemory;

% Get the work memory and delay buffer sizes
workMemorySize = numel(codeWorkMemory);
delayBufferSize = numel(delayBuffer);
fastDelayBufferSize = numel(fastDelayBuffer);

% Set correct data types
frameSize = uint32(frameSize);
numChannels = uint32(numChannels);
delayChain = uint32(delayChain);
workMemorySize = uint32(workMemorySize);
delayBufferSize = uint32(delayBufferSize);
fastDelayBufferSize = uint32(fastDelayBufferSize);
    
y = pool_delay_mdma_init(u, delayBuffer, delayBufferSize, ...
                         fastDelayBuffer, fastDelayBufferSize, ...
                         delayChain, numChannels, frameSize, ...
                         codeWorkMemory, workMemorySize);
    
    % NOTE: The CRL mechanism requires an output for the function call,
    % and appears to be optimized out if that return value isn't used. 
    % This is a dummy operation to make sure CRL ends up in generated code
    codeWorkMemory(1) = y; 

end


% Pool delay CRL MDMA initialization function conceptual specification
function y = pool_delay_mdma_init(u, delayBuffer, delayBufferSize, ...
                                  fastDelayBuffer, fastDelayBufferSize, ...
                                  delayChain, numChannels, frameSize, ...
                                  workMemory, workMemorySize) 
% If target == codegen, error out if no CRL found
coder.replace('-errorifnoreplacement');

% No init simulation code, but need to do something to ensure CRL does not
% get optimized out
y = single(workMemory(1) + 1);

end

== matlab function DelayLibraryBtc/PoolDelay/PoolDelay/Generic/pool delay process ==
  data: u input; delayChain input; y output; fastDelayBuffer data_store_memory
function y = pool_delay_process(u, delayChain)
% Pool delay function provides delay lines for N channels.
%
% Parameters:
%   u:              Input channels [frame size x number of inputs]
%   delayChain:     Delay in samples for each channel [1 x delay per channel]
%
% Global parameters:
%   fastDelayBuffer: Fast delay line circular buffer containing all channel  
%                    delay state data

global fastDelayBuffer;


% Get the fast delay buffer sizes
fastDelayBufferSize = numel(fastDelayBuffer);

% Set correct data types
delayChain = uint32(delayChain);
fastDelayBufferSize = uint32(fastDelayBufferSize);

% Simulation
if(coder.target('MATLAB') || coder.target('Sfun')) 
        y = PoolDelaySim(u, delayChain, fastDelayBufferSize); 
else
        y = PoolDelayCodeGen(u, delayChain, fastDelayBufferSize);
end

end

== matlab function DelayLibraryBtc/PoolDelay/PoolDelay/L2Memory/pool delay process ==
  data: u input; delayChain input; y output; codeWorkMemory data_store_memory; delayBuffer data_store_memory; fastDelayBuffer data_store_memory
function y = pool_delay_process(u, delayChain)
% Pool delay function provides delay lines for N channels. MDMA
% implementation provides integer value delays of a frame or greater. 
%
% Parameters:
%   u:              Input channels [frame size x number of inputs]
%   delayChain:     Delay in samples for each channel [1 x delay per channel]
%
% Global parameters:
%   delayBuffer:     Delay line circular buffer containing all channel  
%                    delay state data
%   fastDelayBuffer: Fast delay line circular buffer containing all channel  
%                    delay state data
%   codeWorkMemory:  Working memory set up during roommode reset/init CRL
%                    function call [1 x codeWorkMemorySize]

global delayBuffer;
global fastDelayBuffer;
global codeWorkMemory;

% Get the fast delay buffer sizes
delayBufferSize = numel(delayBuffer);
fastDelayBufferSize = numel(fastDelayBuffer);

% Set correct data types
delayChain = uint32(delayChain);
delayBufferSize = uint32(delayBufferSize);
fastDelayBufferSize = uint32(fastDelayBufferSize);

% Simulation
if(coder.target('MATLAB') || coder.target('Sfun')) 
        % Simulation does not distribute delay state across two delay
        % buffers. It uses one delay buffer.
        y = PoolDelaySim(u, delayChain, ...
                         (fastDelayBufferSize + delayBufferSize));  
else
        y = pool_delay_mdma_process(u, delayChain, codeWorkMemory);
end
end

% Pool delay CRL MDMA step/process function conceptual specification
function y = pool_delay_mdma_process(u, delayChain, workMemory)
% If target == codegen, error out if no CRL found
coder.replace('-errorifnoreplacement');

[frameSize, numChannels] = size(u);
y = single(zeros(frameSize, numChannels));
end
